simulink model "Temp_controlPlantTest"  (R2016b)
settings: Solver=FixedStepAuto  StartTime=0.0  StopTime=20000  FixedStep=0.05  RelTol=1e-3  EnableMultiTasking=on
undefined symbols (not defined in the file or in its folder): DiscIntNeverNeededParam
libraries: EEE481Arduino x3
settings Model: SimulationMode=external  ExtModeTrigDuration=2  Creator=EliteBook 8470p  LastModifiedBy=rsjoshi1
settings OptimizationCC: LifeSpan=1  MaxStackSize=64
settings DebuggingCC: SFUnexpectedBacktrackingDiag=warning  SFNoUnconditionalDefaultTransitionDiag=warning  SFExecutionAtInitializationDiag=none
settings HardwareCC: ProdBitPerPointer=32  ProdBitPerSizeT=32  ProdBitPerPtrDiffT=32  ProdLargestAtomicInteger=Long  ProdLargestAtomicFloat=Double  ProdWordSize=32  ProdHWDeviceType=ARM Compatible->ARM Cortex
settings RTWCC: SystemTargetFile=ert.tlc  HardwareBoard=Arduino Due  TLCOptions=-aInlineSetEventsForThisBaseRateFcn=TLC_FALSE -aSuppressMultiTaskScheduler=TLC_FALSE -aRateBasedStepFcn=1  TemplateMakefile=ert_default_tmf  Description=Embedded Coder  GenerateReport=on  Toolchain=Arduino ARM v1.6.7  BuildConfiguration=Faster Runs  IncludeHyperlinkInReport=on  LaunchReport=on  GenerateTraceInfo=on  GenerateTraceReport=on  GenerateTraceReportSl=on  GenerateTraceReportSf=on  GenerateTraceReportEml=on
settings CodeAppCC: ForceParamTrailComments=on  IgnoreCustomStorageClasses=off  OperatorAnnotations=on  SimulinkDataObjDesc=on  SFDataObjDesc=on  MATLABFcnDesc=on  InsertBlockDesc=on  MATLABSourceComments=on
settings ERTTargetCC: SupportContinuousTime=on  SupportVariableSizeSignals=on
settings ConfigComp: CovMetricSettings=dw  CovHtmlReporting=on  CovSaveCumulativeToWorkspaceVar=on  CovSaveSingleToWorkspaceVar=on  CovExternalEMLEnable=off

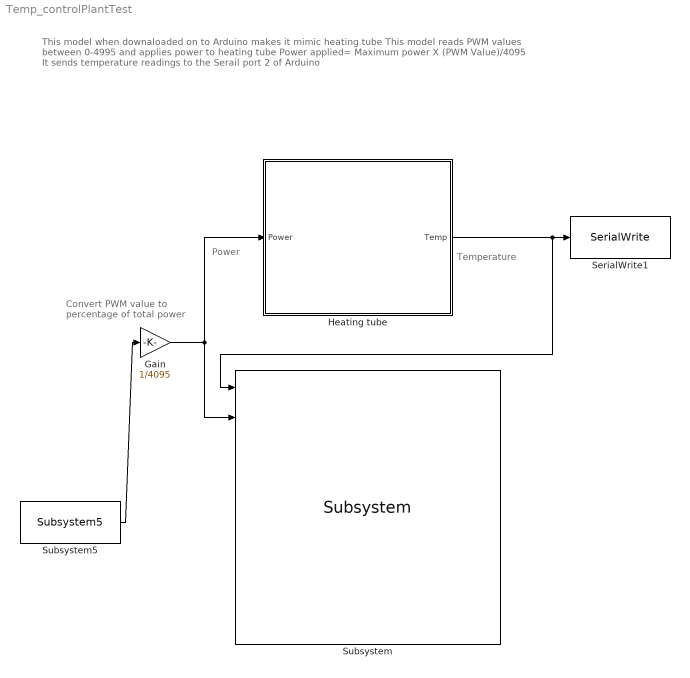
== system Temp_controlPlantTest ==
  note: This model when downaloaded on to Arduino makes it mimic heating tube
      | This model reads PWM values between 0-4995 and applies power to heating tube
      | Power applied= Maximum power X (PWM Value)/4095
      | It sends temperature readings to the Serail port 2 of Arduino
  note: Convert PWM value to
      | percentage of total power
  note: Power
  note: Temperature
  Gain : Gain  Gain=1/4095
  Heating tube : Subsystem
      mask Display: disp('Heating Tube')
  SerialWrite1 : EEE481Arduino/SerialWrite  serialNum=2  Tsa=Tsa
  Subsystem : EEE481Arduino/Subsystem  Tsa=1  rate=0  per=0
  Subsystem5 : EEE481Arduino/Subsystem5  Tsa=Tsa
  wires:
  ? -> ?
  Heating tube/1(Temp) -> SerialWrite1/1, Subsystem/1
  Gain/1 -> Subsystem/2, Heating tube/1(Power)
  Subsystem5/1 -> Gain/1

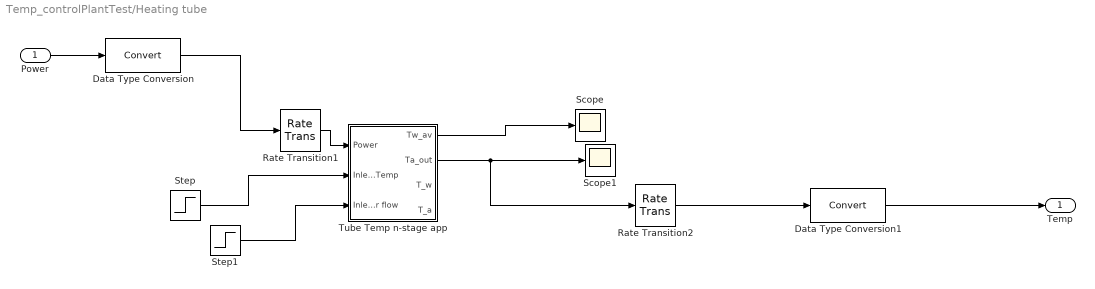
== system Temp_controlPlantTest/Heating tube ==
  Power : Inport
  Data Type Conversion : DataTypeConversion
  Data Type Conversion1 : DataTypeConversion
  Rate Transition1 : RateTransition  OutPortSampleTime=0.05
  Rate Transition2 : RateTransition  OutPortSampleTime=1
  Scope : Scope
  Scope1 : Scope
  Step : Step  Time=10000  Before=25  After=25  SampleTime=0.05
  Step1 : Step  Time=5000  Before=1  SampleTime=0.05
  Tube Temp n-stage app : Subsystem  mask{L=1, n=10, ra=.1, T_01=800, T_a01=25, T_amb=25}
      mask prompts: L "Tube Length"; n "Number of sections"; ra "Tube inner radius"; T_01 "Initial tube temp"; T_a01 "Initial air temp"; T_amb "Ambient Temp"
      mask init:
      | cp=1078;cpa=1134;rhoa=0.5;hs=5;ha=30;rhos=2500;k=2;
      | d=.01;vt=pi*L*((ra+d)*(ra+d)-ra*ra);m=vt*rhos;
      | As=2*pi*(ra+.1)*L;V=pi*ra*ra*L;Aa=2*pi*ra*L;
      | A_d=pi*((ra+d)*(ra+d)-ra*ra);A_rat=1;Li=L/n;
      | T_0=T_01*ones(n,1);T_a0=T_a01*ones(n,1);
  Temp : Outport
  wires:
  Step1/1 -> Tube Temp n-stage app/3(Inlet Air flow)
  Step/1 -> Tube Temp n-stage app/2(Inlet Air Temp)
  Tube Temp n-stage app/2(Ta_out) -> Rate Transition2/1, Scope1/1
  Tube Temp n-stage app/1(Tw_av) -> Scope/1
  Rate Transition1/1 -> Tube Temp n-stage app/1(Power)
  Rate Transition2/1 -> Data Type Conversion1/1
  Power/1 -> Data Type Conversion/1
  Data Type Conversion/1 -> Rate Transition1/1
  Data Type Conversion1/1 -> Temp/1

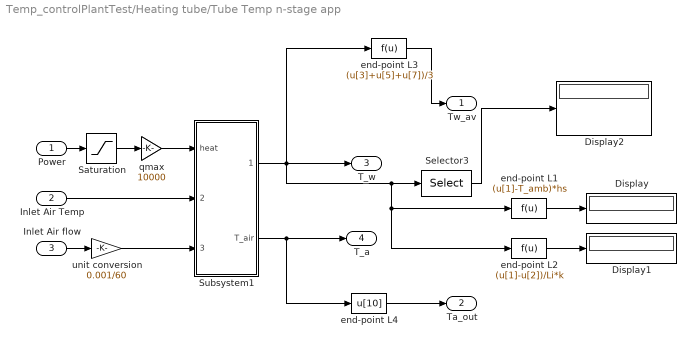
== system Temp_controlPlantTest/Heating tube/Tube Temp n-stage app ==
  Power : Inport
  Inlet Air Temp : Inport  Port=2
  Inlet Air flow : Inport  Port=3
  Display : Display
      settings: Format=short_e
  Display1 : Display
      settings: Format=short_e
  Display2 : Display
      settings: Format=short_e
  Saturation : Saturate  UpperLimit=1  LowerLimit=0
  Selector3 : Selector  InputPortWidth=n  IndexOptions=Index vector (dialog)  Indices=[1,2]  OutputSizes=1
  Subsystem1 : Subsystem
  end-point L1 : Fcn  Expr=(u[1]-T_amb)*hs
  end-point L2 : Fcn  Expr=(u[1]-u[2])/Li*k
  end-point L3 : Fcn  Expr=(u[3]+u[5]+u[7])/3
  end-point L4 : Fcn  Expr=u[10]
  qmax : Gain  Gain=10000  SaturateOnIntegerOverflow=on  OutDataTypeStr=Inherit: Same as input  ParamDataTypeStr=Inherit: Same as input
  unit conversion : Gain  Gain=0.001/60  SaturateOnIntegerOverflow=on  OutDataTypeStr=Inherit: Same as input  ParamDataTypeStr=Inherit: Same as input
  Tw_av : Outport
  Ta_out : Outport  Port=2
  T_w : Outport  Port=3
  T_a : Outport  Port=4
  wires:
  end-point L2/1 -> Display1/1
  end-point L1/1 -> Display/1
  Selector3/1 -> Display2/1
  Subsystem1/2(T_air) -> end-point L4/1, T_a/1
  Subsystem1/1(T_wall) -> end-point L3/1, end-point L2/1, end-point L1/1, Selector3/1, T_w/1
  unit conversion/1 -> Subsystem1/3(Air flow)
  Inlet Air flow/1 -> unit conversion/1
  Power/1 -> Saturation/1
  Saturation/1 -> qmax/1
  Inlet Air Temp/1 -> Subsystem1/2(T_a_inlet)
  qmax/1 -> Subsystem1/1(heat)
  end-point L3/1 -> Tw_av/1
  end-point L4/1 -> Ta_out/1

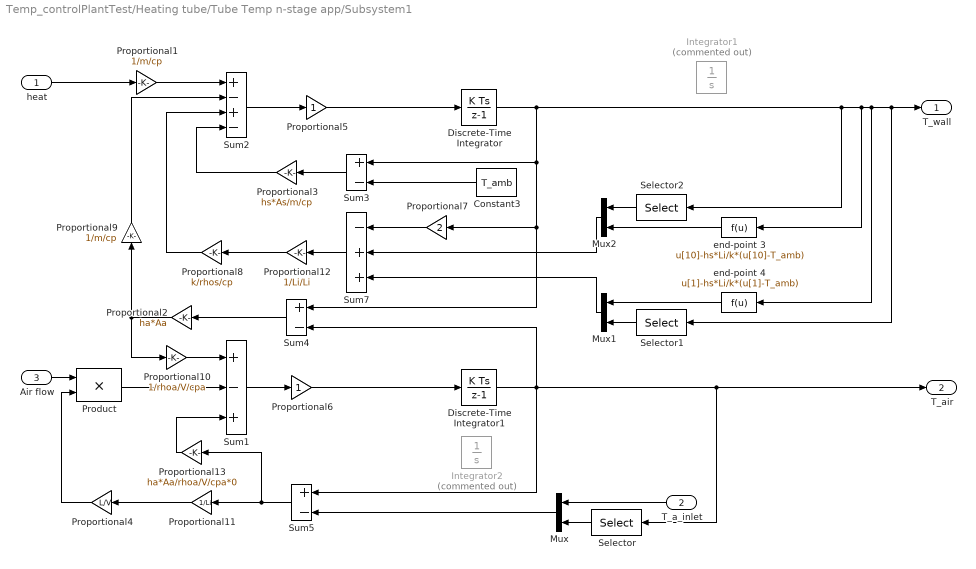
== system Temp_controlPlantTest/Heating tube/Tube Temp n-stage app/Subsystem1 ==
  heat : Inport
  T_a_inlet : Inport  Port=2
  Air flow : Inport  Port=3
  Constant3 : Constant  Value=T_amb
  Discrete-Time Integrator : DiscreteIntegrator  InitialCondition=T_0  InitialConditionSetting=State (most efficient)  SampleTime=0.05  ICPrevOutput=DiscIntNeverNeededParam  ICPrevScaledInput=DiscIntNeverNeededParam
  Discrete-Time Integrator1 : DiscreteIntegrator  InitialCondition=T_a0  InitialConditionSetting=State (most efficient)  SampleTime=0.05  ICPrevOutput=DiscIntNeverNeededParam  ICPrevScaledInput=DiscIntNeverNeededParam
  Integrator1 : Integrator  Commented=on  InitialCondition=T_0
  Integrator2 : Integrator  Commented=on  InitialCondition=T_a0
  Mux : Mux  Inputs=2
  Mux1 : Mux  Inputs=2
  Mux2 : Mux  Inputs=2
  Product : Product  SaturateOnIntegerOverflow=on  RndMeth=Zero  InputSameDT=on  OutDataTypeStr=Inherit: Same as first input
  Proportional1 : Gain  Gain=1/m/cp  SaturateOnIntegerOverflow=on  OutDataTypeStr=Inherit: Same as input  ParamDataTypeStr=Inherit: Same as input
  Proportional10 : Gain  Gain=1/rhoa/V/cpa  SaturateOnIntegerOverflow=on  OutDataTypeStr=Inherit: Same as input  ParamDataTypeStr=Inherit: Same as input
  Proportional11 : Gain  Gain=1/Li  SaturateOnIntegerOverflow=on  OutDataTypeStr=Inherit: Same as input  ParamDataTypeStr=Inherit: Same as input
  Proportional12 : Gain  Gain=1/Li/Li  SaturateOnIntegerOverflow=on  OutDataTypeStr=Inherit: Same as input  ParamDataTypeStr=Inherit: Same as input
  Proportional13 : Gain  Gain=ha*Aa/rhoa/V/cpa*0  SaturateOnIntegerOverflow=on  OutDataTypeStr=Inherit: Same as input  ParamDataTypeStr=Inherit: Same as input
  Proportional2 : Gain  Gain=ha*Aa  SaturateOnIntegerOverflow=on  OutDataTypeStr=Inherit: Same as input  ParamDataTypeStr=Inherit: Same as input
  Proportional3 : Gain  Gain=hs*As/m/cp  SaturateOnIntegerOverflow=on  OutDataTypeStr=Inherit: Same as input  ParamDataTypeStr=Inherit: Same as input
  Proportional4 : Gain  Gain=L/V  SaturateOnIntegerOverflow=on  OutDataTypeStr=Inherit: Same as input  ParamDataTypeStr=Inherit: Same as input
  Proportional5 : Gain  SaturateOnIntegerOverflow=on  OutDataTypeStr=Inherit: Same as input  ParamDataTypeStr=Inherit: Same as input
  Proportional6 : Gain  SaturateOnIntegerOverflow=on  OutDataTypeStr=Inherit: Same as input  ParamDataTypeStr=Inherit: Same as input
  Proportional7 : Gain  Gain=2  SaturateOnIntegerOverflow=on  OutDataTypeStr=Inherit: Same as input  ParamDataTypeStr=Inherit: Same as input
  Proportional8 : Gain  Gain=k/rhos/cp  SaturateOnIntegerOverflow=on  OutDataTypeStr=Inherit: Same as input  ParamDataTypeStr=Inherit: Same as input
  Proportional9 : Gain  Gain=1/m/cp  SaturateOnIntegerOverflow=on  OutDataTypeStr=Inherit: Same as input  ParamDataTypeStr=Inherit: Same as input
  Selector : Selector  InputPortWidth=n  IndexOptions=Index vector (dialog)  Indices=[1:n-1]  OutputSizes=1
  Selector1 : Selector  InputPortWidth=n  IndexOptions=Index vector (dialog)  Indices=[1:n-1]  OutputSizes=1
  Selector2 : Selector  InputPortWidth=n  IndexOptions=Index vector (dialog)  Indices=[2:n]  OutputSizes=1
  Sum1 : Sum  Inputs=+-+  SaturateOnIntegerOverflow=on  InputSameDT=on  OutDataTypeStr=Inherit: Same as first input
  Sum2 : Sum  Inputs=+-+-  SaturateOnIntegerOverflow=on  InputSameDT=on  OutDataTypeStr=Inherit: Same as first input
  Sum3 : Sum  Inputs=+-  SaturateOnIntegerOverflow=on  InputSameDT=on  OutDataTypeStr=Inherit: Same as first input
  Sum4 : Sum  Inputs=+-  SaturateOnIntegerOverflow=on  InputSameDT=on  OutDataTypeStr=Inherit: Same as first input
  Sum5 : Sum  Inputs=+-  SaturateOnIntegerOverflow=on  InputSameDT=on  OutDataTypeStr=Inherit: Same as first input
  Sum7 : Sum  Inputs=-++  SaturateOnIntegerOverflow=on  InputSameDT=on  OutDataTypeStr=Inherit: Same as first input
  end-point 3 : Fcn  Expr=u[10]-hs*Li/k*(u[10]-T_amb)
  end-point 4 : Fcn  Expr=u[1]-hs*Li/k*(u[1]-T_amb)
  T_wall : Outport
  T_air : Outport  Port=2
  wires:
  Proportional5/1 -> Discrete-Time Integrator/1
  Proportional3/1 -> Sum2/4
  Proportional13/1 -> Sum1/3
  end-point 3/1 -> Mux2/2
  end-point 4/1 -> Mux1/1
  Selector2/1 -> Mux2/1
  Selector1/1 -> Mux1/2
  Mux/1 -> Sum5/2
  Selector/1 -> Mux/2
  T_a_inlet/1 -> Mux/1
  Air flow/1 -> Product/1
  Product/1 -> Sum1/2
  Proportional4/1 -> Product/2
  Proportional12/1 -> Proportional8/1
  Proportional11/1 -> Proportional4/1
  Proportional10/1 -> Sum1/1
  Proportional9/1 -> Sum2/2
  Proportional1/1 -> Sum2/1
  Sum2/1 -> Proportional5/1
  Discrete-Time Integrator/1 -> end-point 3/1, end-point 4/1, Selector1/1, T_wall/1, Selector2/1, Sum3/1, Sum4/1, Proportional7/1
  Constant3/1 -> Sum3/2
  Sum3/1 -> Proportional3/1
  Sum4/1 -> Proportional2/1
  Proportional2/1 -> Proportional10/1, Proportional9/1
  Sum1/1 -> Proportional6/1
  Discrete-Time Integrator1/1 -> T_air/1, Selector/1, Sum4/2, Sum5/1
  Sum5/1 -> Proportional13/1, Proportional11/1
  heat/1 -> Proportional1/1
  Proportional6/1 -> Discrete-Time Integrator1/1
  Proportional7/1 -> Sum7/1
  Mux2/1 -> Sum7/2
  Mux1/1 -> Sum7/3
  Sum7/1 -> Proportional12/1
  Proportional8/1 -> Sum2/3
